simulink model "accNoiseStudy"  (R2017b)
settings: Solver=VariableStepAuto  StartTime=0.0  StopTime=time(end)  RelTol=1e-3
undefined symbols (not defined in the file): ST
settings Model: Creator=CC  LastModifiedBy=CC

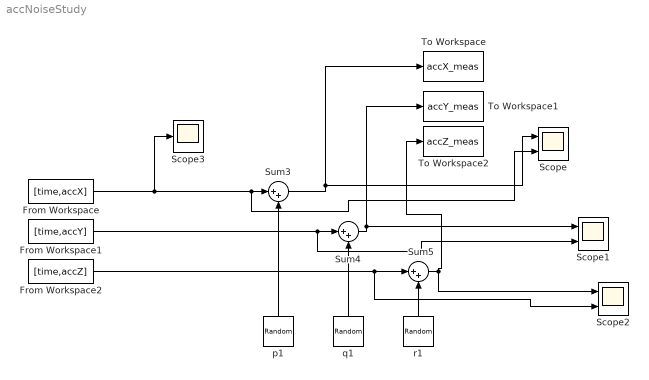
== system accNoiseStudy ==
  From Workspace : FromWorkspace  VariableName=[time,accX]  SampleTime=0
  From Workspace1 : FromWorkspace  VariableName=[time,accY]  SampleTime=0
  From Workspace2 : FromWorkspace  VariableName=[time,accZ]  SampleTime=0
  Scope : Scope  NumInputPorts=2
  Scope1 : Scope  NumInputPorts=2
  Scope2 : Scope  NumInputPorts=2
  Scope3 : Scope
  Sum3 : Sum  Inputs=|++
  Sum4 : Sum  Inputs=|++
  Sum5 : Sum  Inputs=|++
  To Workspace : ToWorkspace  VariableName=accX_meas  SampleTime=-1
  To Workspace1 : ToWorkspace  VariableName=accY_meas  SampleTime=-1
  To Workspace2 : ToWorkspace  VariableName=accZ_meas  SampleTime=-1
  p1 : RandomNumber  Variance=0.01  SampleTime=ST
  q1 : RandomNumber  Variance=0.01  SampleTime=ST
  r1 : RandomNumber  Variance=0.01  SampleTime=ST
  wires:
  r1/1 -> Sum5/2
  q1/1 -> Sum4/2
  p1/1 -> Sum3/2
  From Workspace/1 -> Scope3/1, Scope/2, Sum3/1
  From Workspace1/1 -> Scope1/2, Sum4/1
  From Workspace2/1 -> Scope2/2, Sum5/1
  Sum3/1 -> To Workspace/1, Scope/1
  Sum4/1 -> To Workspace1/1, Scope1/1
  Sum5/1 -> To Workspace2/1, Scope2/1
